simulink model "model01_nc"  (R2021a)
settings: Solver=VariableStepAuto  StartTime=0  StopTime=tf  RelTol=1e-3
values from neighbouring files (symbols this model uses):
  AR_state_real = 0    [model01_simulation_loop.m]
  area = 0.01    [create_p.mat]    (also in create_params.m; model01_simulation_loop.m = 150)
  C = crop_params.C    [model01_simulation_loop.m]
  clima = clima_fcn(posixtime(dat_time))    [model01_simulation_loop.m]    (also in model_compile.m = [273.15+10 400 50 0.1])
  l_w = 0.01    [create_p.mat]    (also in create_params.m; model01_simulation_loop.m)
  lamb_s = 2    [create_p.mat]    (also in create_params.m; model01_simulation_loop.m)
  maxPower = 70000    [create_p.mat]    (also in create_params.m)
  N = crop_params.N    [model01_simulation_loop.m]
  PID_p = 70000    [create_p.mat]    (also in create_params.m)
  R = crop_params.R    [model01_simulation_loop.m]
  set_point_Ti = 16.5    [create_p.mat]    (also in create_params.m)
undefined symbols (not defined in the file or in its folder): Qreal
libraries: HORTISIM x9
settings Model: SimulationMode=accelerator  OrderedModelArguments=off  Creator=djoroya  LastModifiedBy=djoroya
settings DataIOCC: SaveFormat=StructureWithTime
settings OptimizationCC: EfficientMapNaN2IntZero=off
settings DebuggingCC: UnconnectedInputMsg=none  UnconnectedOutputMsg=none  UnconnectedLineMsg=none
settings HardwareCC: TargetBitPerLong=64  TargetBitPerPointer=64  TargetBitPerSizeT=64  TargetBitPerPtrDiffT=64  TargetLongLongMode=on  TargetIntDivRoundTo=Zero  TargetEndianess=LittleEndian  TargetWordSize=64  TargetHWDeviceType=MATLAB Host  ProdEqTarget=off
settings CodeAppCC: MaxIdLength=128
settings GRTTargetCC: CombineOutputUpdateFcns=off  GRTInterface=on

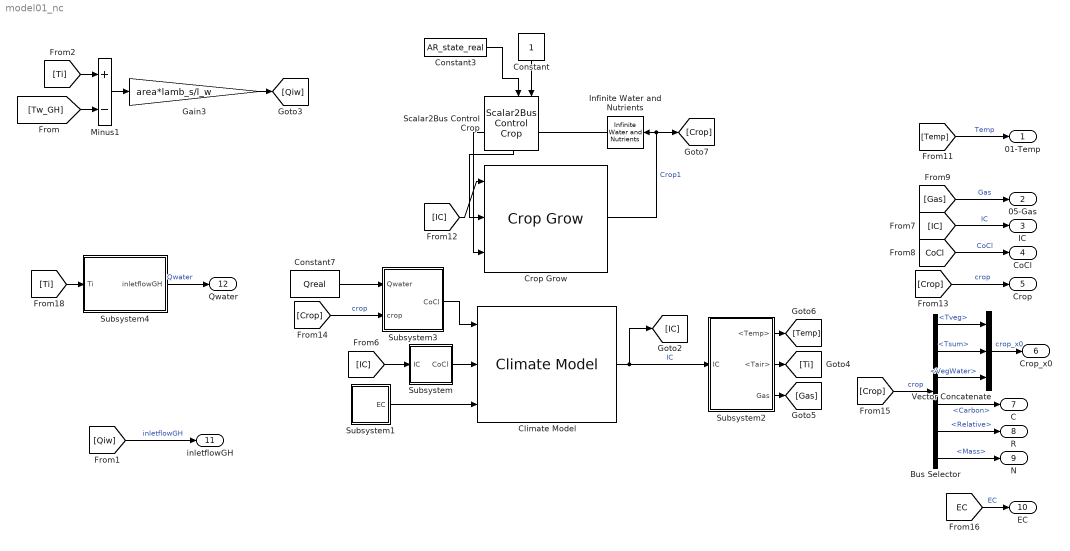
== system model01_nc ==
  Bus Selector : BusSelector  OutputSignals=HeatVars.Tveg,Tsum,Water.WaterState.VegWater,Carbon,Relative,Nutrients.Mass
  Climate Model : HORTISIM/Climate/Models/Climate Model  hour0=hour0  G0=G0  T0=T0  H=climate_GH3.H  A_f=climate_GH3.A_f  A_c=climate_GH3.A_c  minWindows=climate_GH3.minWindows  lam_s=climate_GH3.lam_s  c_s=climate_GH3.c_s  l_s=climate_GH3.l_s  rhod_s=climate_GH3.rhod_s  int_air_speed=climate_GH3.int_air_speed  alpha_i=climate_GH3.alpha_i  alpha_c=climate_GH3.alpha_c  tau_c=climate_GH3.tau_c  alpha_f=climate_GH3.alpha_f  d_c=climate_GH3.d_c  cd_c=climate_GH3.cd_c  T_ss=climate_GH3.T_ss
      settings: SourceProductName=Horti Simulator
  Constant : Constant
  Constant3 : Constant  Value=AR_state_real
  Constant7 : Constant  Value=Qreal
  Crop Grow : HORTISIM/Horticulture/Models/Crop Grow  Chi_nutrients=crop_params.Chi_nutrients  A_v=crop_params.A_v  plants_density=crop_params.plants_density  fraction_DM=crop_params.fraction_DM  min_water_capacity=crop_params.min_water_capacity  C_buf_max=crop_params.C_buf_max  T_v_start_fruit=crop_params.T_v_start_fruit  int_air_speed=crop_params.int_air_speed  b_N_uptake=crop_params.b_N_uptake  Tv=Tv  C=C  R=R  Tsum=Tsum  C_wv=C_wv  N=N  rg_fruit=crop_params.rg_fruit  c_fruit_m=crop_params.c_fruit_m  c_fruit_g=crop_params.c_fruit_g  rg_leaf=crop_params.rg_leaf  c_leaf_m=crop_params.c_leaf_m  c_leaf_g=crop_params.c_leaf_g  rg_stem=crop_params.rg_stem  c_stem_m=crop_params.c_stem_m  c_stem_g=crop_params.c_stem_g  VelocityAbsortion=crop_params.VelocityAbsortion  T_max_v=crop_params.T_max_v  s_max_T=crop_params.s_max_T  s_min_T=crop_params.s_min_T  s_buforg_buf=crop_params.s_buforg_buf  T_sum_end=crop_params.T_sum_end  T_max_v24=crop_params.T_max_v24  T_min_v24=crop_params.T_min_v24  s_min_T24=crop_params.s_min_T24  s_max_T24=crop_params.s_max_T24  T_min_v=crop_params.T_min_v
      settings: SourceProductName=Horti Simulator
  Gain3 : Gain  Gain=area*lamb_s/l_w
  Infinite Water and Nutrients : HORTISIM/Other  Functions/Infinite Water and Nutrients  SystemSampleTime=-1  VariantActivationTime=update diagram  Latency=0  AutoFrameSizeCalculation=off
      settings: SourceProductName=Horti Simulator
  Minus1 : Sum  Inputs=+-
  Scalar2Bus Control Crop : HORTISIM/Other  Functions/Scalar2Bus Control Crop  SystemSampleTime=-1  VariantActivationTime=update diagram  Latency=0  AutoFrameSizeCalculation=off
      settings: SourceProductName=Horti Simulator
  Subsystem : Subsystem
  Subsystem1 : Subsystem
  Subsystem2 : Subsystem
  Subsystem3 : Subsystem
  Subsystem4 : Subsystem
  Vector Concatenate : Concatenate  NumInputs=3
  01-Temp : Outport
  05-Gas : Outport  Port=2
  IC : Outport  Port=3
  CoCl : Outport  Port=4
  Crop : Outport  Port=5
  Crop_x0 : Outport  Port=6
  C : Outport  Port=7
  R : Outport  Port=8
  N : Outport  Port=9
  EC : Outport  Port=10
  inletflowGH : Outport  Port=11
  Qwater : Outport  Port=12
  wires:
  [Tw_GH] -> Minus1/2
  Subsystem/1(CoCl) -> Climate Model/2
  [Ti] -> Minus1/1
  Minus1/1 -> Gain3/1
  Climate Model/1 -> [IC], Subsystem2/1(IC)  "IC"
  Gain3/1 -> [Qiw]
  Subsystem1/1(EC) -> Climate Model/3
  [IC] -> Subsystem/1(IC)
  [IC] -> IC/1  "IC"
  [CoCl] -> CoCl/1  "CoCl"
  [Gas] -> 05-Gas/1  "Gas"
  [Temp] -> 01-Temp/1  "Temp"
  Infinite Water and Nutrients/1 -> Crop Grow/3
  Crop Grow/1 -> [Crop], Infinite Water and Nutrients/1  "Crop1"
  Subsystem2/1(<Temp>) -> [Temp]
  Subsystem2/2(<Tair>) -> [Ti]
  Subsystem2/3(Gas) -> [Gas]
  [IC] -> Crop Grow/1
  [Crop] -> Crop/1  "crop"
  [Crop] -> Subsystem3/2(crop)  "crop"
  Subsystem3/1(CoCl) -> Climate Model/1
  Scalar2Bus Control Crop/1 -> Crop Grow/2
  Constant/1 -> Scalar2Bus Control Crop/4
  Constant3/1 -> Scalar2Bus Control Crop/3
  [Crop] -> Bus Selector/1  "crop"
  Bus Selector/2 -> Vector Concatenate/2  "<Tsum>"
  Bus Selector/3 -> Vector Concatenate/3  "<VegWater>"
  Bus Selector/1 -> Vector Concatenate/1  "<Tveg>"
  Vector Concatenate/1 -> Crop_x0/1  "crop_x0"
  Bus Selector/4 -> C/1  "<Carbon>"
  Bus Selector/5 -> R/1  "<Relative>"
  Bus Selector/6 -> N/1  "<Mass>"
  [EC] -> EC/1  "EC"
  Subsystem4/1(inletflowGH) -> Qwater/1  "Qwater"
  [Ti] -> Subsystem4/1(Ti)
  [Qiw] -> inletflowGH/1  "inletflowGH"
  Constant7/1 -> Subsystem3/1(Qwater)

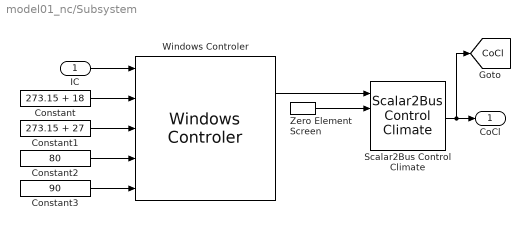
== system model01_nc/Subsystem ==
  IC : Inport
  Constant : Constant  Value=273.15 + 18
  Constant1 : Constant  Value=273.15 + 27
  Constant2 : Constant  Value=80
  Constant3 : Constant  Value=90
  Scalar2Bus Control Climate : HORTISIM/Other  Functions/Scalar2Bus  Control Climate  SystemSampleTime=-1  VariantActivationTime=update diagram  Latency=0  AutoFrameSizeCalculation=off
      settings: SourceProductName=Horti Simulator
  Windows Controler : HORTISIM/Climate/Controls/Windows Controler  Power=100  max_night=10  tau=600  RadThreshold=10  AR=10
      settings: SourceProductName=Horti Simulator
  Zero Element Screen : HORTISIM/Other  Functions/Zero Element Screen  SystemSampleTime=-1  VariantActivationTime=update diagram  Latency=0  AutoFrameSizeCalculation=off
      settings: SourceProductName=Horti Simulator
  CoCl : Outport
  tag scope: CoCl=global
  wires:
  Scalar2Bus Control Climate/1 -> [CoCl], CoCl/1
  Windows Controler/1 -> Scalar2Bus Control Climate/1
  Zero Element Screen/1 -> Scalar2Bus Control Climate/2
  IC/1 -> Windows Controler/1
  Constant/1 -> Windows Controler/2
  Constant1/1 -> Windows Controler/3
  Constant2/1 -> Windows Controler/4
  Constant3/1 -> Windows Controler/5

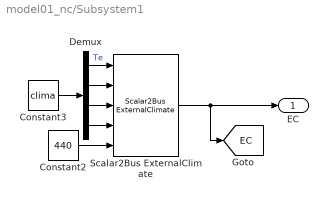
== system model01_nc/Subsystem1 ==
  Constant2 : Constant  Value=440
  Constant3 : Constant  Value=clima
  Demux : Demux
  Scalar2Bus ExternalClimate : HORTISIM/Other  Functions/Scalar2Bus ExternalClimate  SystemSampleTime=-1  VariantActivationTime=update diagram  Latency=0  AutoFrameSizeCalculation=off
      settings: SourceProductName=Horti Simulator
  EC : Outport
  tag scope: EC=global
  wires:
  Constant3/1 -> Demux/1
  Demux/3 -> Scalar2Bus ExternalClimate/3
  Scalar2Bus ExternalClimate/1 -> [EC], EC/1
  Demux/4 -> Scalar2Bus ExternalClimate/4
  Demux/2 -> Scalar2Bus ExternalClimate/2
  Constant2/1 -> Scalar2Bus ExternalClimate/5
  Demux/1 -> Scalar2Bus ExternalClimate/1  "Te"

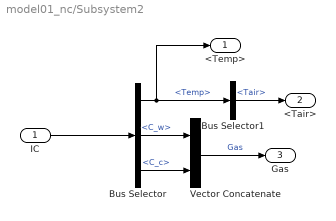
== system model01_nc/Subsystem2 ==
  IC : Inport
  Bus Selector : BusSelector  OutputSignals=Temp,Gas.C_w,Gas.C_c
  Bus Selector1 : BusSelector  OutputSignals=Tair
  Vector Concatenate : Concatenate
  <Temp> : Outport
  <Tair> : Outport  Port=2
  Gas : Outport  Port=3
  wires:
  Bus Selector/1 -> <Temp>/1, Bus Selector1/1  "<Temp>"
  Bus Selector1/1 -> <Tair>/1  "<Tair>"
  Vector Concatenate/1 -> Gas/1  "Gas"
  Bus Selector/3 -> Vector Concatenate/2  "<C_c>"
  IC/1 -> Bus Selector/1
  Bus Selector/2 -> Vector Concatenate/1  "<C_w>"

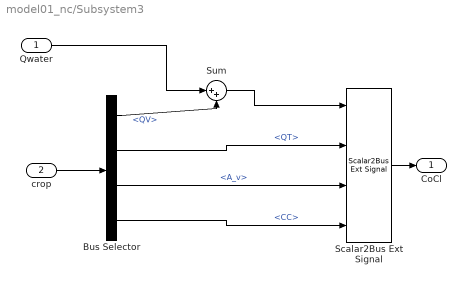
== system model01_nc/Subsystem3 ==
  Qwater : Inport
  crop : Inport  Port=2
  Bus Selector : BusSelector  OutputSignals=HeatVars.QV,HeatVars.QT,A_v,CC
  "Scalar2Bus Ext Signal " : HORTISIM/Other  Functions/Scalar2Bus Ext Signal    SystemSampleTime=-1  VariantActivationTime=update diagram  Latency=0  AutoFrameSizeCalculation=off
      settings: SourceProductName=Horti Simulator
  Sum : Sum  Inputs=|++
  CoCl : Outport
  wires:
  "Scalar2Bus Ext Signal "/1 -> CoCl/1
  Bus Selector/4 -> "Scalar2Bus Ext Signal "/4  "<CC>"
  Sum/1 -> "Scalar2Bus Ext Signal "/1
  Qwater/1 -> Sum/1
  crop/1 -> Bus Selector/1
  Bus Selector/1 -> Sum/2  "<QV>"
  Bus Selector/2 -> "Scalar2Bus Ext Signal "/2  "<QT>"
  Bus Selector/3 -> "Scalar2Bus Ext Signal "/3  "<A_v>"

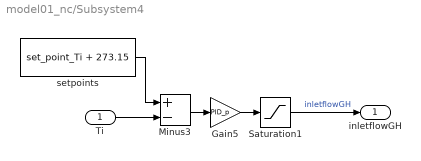
== system model01_nc/Subsystem4 ==
  Ti : Inport
  Gain5 : Gain  Gain=PID_p
  Minus3 : Sum  Inputs=+-
  Saturation1 : Saturate  UpperLimit=maxPower  LowerLimit=0
  setpoints : Constant  Value=set_point_Ti + 273.15
  inletflowGH : Outport
  wires:
  Saturation1/1 -> inletflowGH/1  "inletflowGH"
  Ti/1 -> Minus3/2
  Gain5/1 -> Saturation1/1
  Minus3/1 -> Gain5/1
  setpoints/1 -> Minus3/1
